simulink model "GridFormingConverter"  (R2024b)
settings: Solver=ode1be  StartTime=0.0  StopTime=simulationTime  FixedStep=gridInverter.vsm.samplingTime  MaxStep=gridInverter.vsm.samplingTime  RelTol=1e-3  AbsTol=1e-3
PreLoadFcn:
  | % Parameterize the model
  | GridFormingConverterInputParameters;
  | GFLParameters;
PostLoadFcn:
  | GridFormingConverterTestCondition;
  | GFLParameters;
undefined symbols (not defined in the file or in its folder): base, ConvCtrl, ConvPlt, DiscIntNeverNeededParam, Discrete, Fault, gcbh, GFMGFLSelect, grid, gridInverter, HMI, localSolverSampleTime, magnitude, PlantSim, scrFactorRg, scrFactorXg, sps, sps_rtmsupport, spsPLL3phModel, transformer, TransmissionLine, Trf
libraries: powerlib_extras x39, ee_lib x21, eeGeneralControl x19, nesl_utility x16, simulink x13, eeTransforms x10, fl_lib x7, spsSecondOrderFilterLib x4, spsabctodq0Lib x4, spsPower3phInstantaneousLib x3, spsMeanLib x2, eeSinGeneratorThreePhase x1
(part 4 of 6)

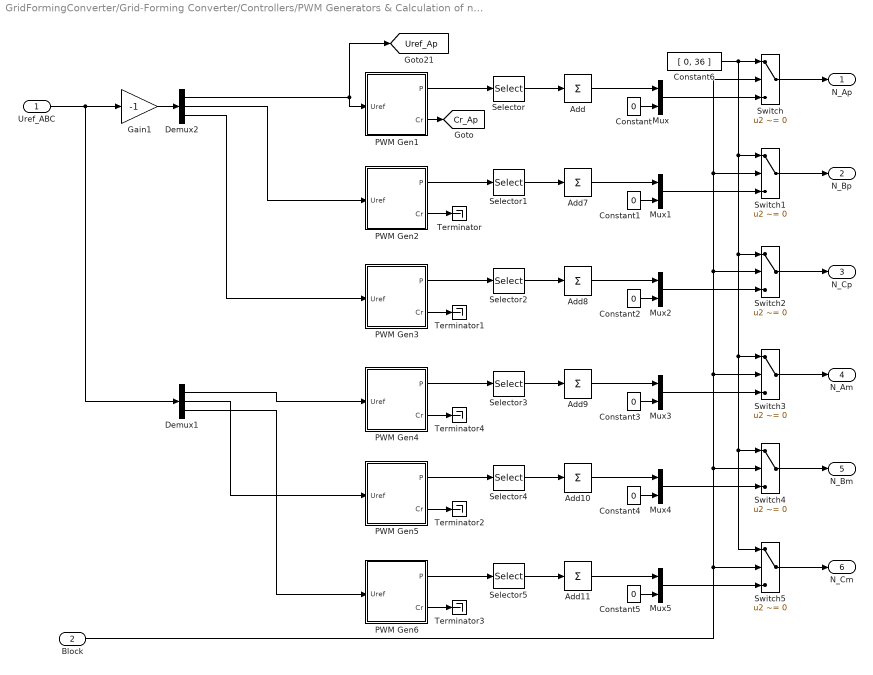
== system GridFormingConverter/Grid-Forming Converter/Controllers/PWM Generators & Calculation of number of inserted modules (Nin) and number of blocked module (Nbl) ==
  Uref_ABC : Inport  PortDimensions=3
  Block : Inport  Port=2
  Add{,7..11} (6 alike) : Sum  Inputs=1
  Constant{,1..5} (6 alike) : Constant  Value=0
  Constant6 : Constant  Value=[ 0, 36 ]
  Demux1 : Demux  Outputs=3
  Demux2 : Demux  Outputs=3
  Gain1 : Gain  Gain=-1
  Mux{,1..5} (6 alike) : Mux  Inputs=2
  PWM Gen1 : Subsystem  mask(PWM generator for half-bridge MMC){n=ConvPlt.Nb_PM, Fc=ConvPlt.Fc, Ts=PlantSim.Ts}
      mask prompts: n "Number of half-bridges"; Fc "Carriers frequency (Hz)"; Ts "Sample time (s)"
      mask init:
      | Tc=1/Fc;
      |         Pc= [ 0:360/n:360-360/n]*pi/180;
      |         Offset=Pc/(2*pi);
      |         Offset_Cr=Pc/(2*pi)*Tc;
      |         p=0;
      |         for m=1:2:2*n
      |             p=p+1;
      |             SelectPulsesPS(m)=p;
      |             SelectPulsesPS(m+1)=p+n;
      |         end
  PWM Gen2 : Subsystem  mask(PWM generator for half-bridge MMC){n=ConvPlt.Nb_PM, Fc=ConvPlt.Fc, Ts=PlantSim.Ts}
      mask prompts: n "Number of half-bridges"; Fc "Carriers frequency (Hz)"; Ts "Sample time (s)"
      mask init: same as GridFormingConverter/Grid-Forming Converter/Controllers/PWM Generators & Calculation of number of inserted modules (Nin) and number of blocked module (Nbl)/PWM Gen1
  PWM Gen3 : Subsystem  mask(PWM generator for half-bridge MMC){n=ConvPlt.Nb_PM, Fc=ConvPlt.Fc, Ts=PlantSim.Ts}
      mask prompts: n "Number of half-bridges"; Fc "Carriers frequency (Hz)"; Ts "Sample time (s)"
      mask init: same as GridFormingConverter/Grid-Forming Converter/Controllers/PWM Generators & Calculation of number of inserted modules (Nin) and number of blocked module (Nbl)/PWM Gen1
  PWM Gen4 : Subsystem  mask(PWM generator for half-bridge MMC){n=ConvPlt.Nb_PM, Fc=ConvPlt.Fc, Ts=PlantSim.Ts}
      mask prompts: n "Number of half-bridges"; Fc "Carriers frequency (Hz)"; Ts "Sample time (s)"
      mask init: same as GridFormingConverter/Grid-Forming Converter/Controllers/PWM Generators & Calculation of number of inserted modules (Nin) and number of blocked module (Nbl)/PWM Gen1
  PWM Gen5 : Subsystem  mask(PWM generator for half-bridge MMC){n=ConvPlt.Nb_PM, Fc=ConvPlt.Fc, Ts=PlantSim.Ts}
      mask prompts: n "Number of half-bridges"; Fc "Carriers frequency (Hz)"; Ts "Sample time (s)"
      mask init: same as GridFormingConverter/Grid-Forming Converter/Controllers/PWM Generators & Calculation of number of inserted modules (Nin) and number of blocked module (Nbl)/PWM Gen1
  PWM Gen6 : Subsystem  mask(PWM generator for half-bridge MMC){n=ConvPlt.Nb_PM, Fc=ConvPlt.Fc, Ts=PlantSim.Ts}
      mask prompts: n "Number of half-bridges"; Fc "Carriers frequency (Hz)"; Ts "Sample time (s)"
      mask init: same as GridFormingConverter/Grid-Forming Converter/Controllers/PWM Generators & Calculation of number of inserted modules (Nin) and number of blocked module (Nbl)/PWM Gen1
  Selector{,1..5} (6 alike) : Selector  InputPortWidth=72  IndexOptions=Index vector (dialog)  Indices=[1:2:71]  OutputSizes=1
  Switch{,1..5} (6 alike) : Switch  Criteria=u2 ~= 0  SaturateOnIntegerOverflow=off  InputSameDT=off
  Terminator{,1..4} (5 alike) : Terminator
  N_Ap : Outport
  N_Bp : Outport  Port=2
  N_Cp : Outport  Port=3
  N_Am : Outport  Port=4
  N_Bm : Outport  Port=5
  N_Cm : Outport  Port=6
  tag scope: Cr_Ap=global, Uref_Ap=global
  wires:
  Demux1/2 -> PWM Gen5/1(Uref)
  Demux1/3 -> PWM Gen6/1(Uref)
  Demux1/1 -> PWM Gen4/1(Uref)
  Demux2/3 -> PWM Gen3/1(Uref)
  PWM Gen1/1(P) -> Selector/1
  PWM Gen2/1(P) -> Selector1/1
  PWM Gen3/1(P) -> Selector2/1
  PWM Gen4/1(P) -> Selector3/1
  PWM Gen5/1(P) -> Selector4/1
  PWM Gen6/1(P) -> Selector5/1
  Mux2/1 -> Switch2/3
  Mux5/1 -> Switch5/3
  Mux4/1 -> Switch4/3
  Mux3/1 -> Switch3/3
  Block/1 -> Switch5/2, Switch4/2, Switch3/2, Switch2/2, Switch1/2, Switch/2
  Add11/1 -> Mux5/1
  Add10/1 -> Mux4/1
  Constant3/1 -> Mux3/2
  Switch5/1 -> N_Cm/1
  Add/1 -> Mux/1
  Switch4/1 -> N_Bm/1
  Switch2/1 -> N_Cp/1
  Constant4/1 -> Mux4/2
  Switch1/1 -> N_Bp/1
  Mux/1 -> Switch/3
  Add8/1 -> Mux2/1
  Add9/1 -> Mux3/1
  Constant2/1 -> Mux2/2
  Constant6/1 -> Switch1/1, Switch2/1, Switch3/1, Switch4/1, Switch5/1, Switch/1
  Mux1/1 -> Switch1/3
  Switch3/1 -> N_Am/1
  Switch/1 -> N_Ap/1
  Constant5/1 -> Mux5/2
  Constant1/1 -> Mux1/2
  Add7/1 -> Mux1/1
  Constant/1 -> Mux/2
  Selector5/1 -> Add11/1
  Selector4/1 -> Add10/1
  Selector3/1 -> Add9/1
  Selector2/1 -> Add8/1
  Selector1/1 -> Add7/1
  Selector/1 -> Add/1
  PWM Gen3/2(Cr) -> Terminator1/1
  PWM Gen1/2(Cr) -> [Cr_Ap]
  Gain1/1 -> Demux2/1
  Demux2/1 -> [Uref_Ap], PWM Gen1/1(Uref)
  Demux2/2 -> PWM Gen2/1(Uref)
  PWM Gen2/2(Cr) -> Terminator/1
  PWM Gen6/2(Cr) -> Terminator3/1
  Uref_ABC/1 -> Demux1/1, Gain1/1
  PWM Gen5/2(Cr) -> Terminator2/1
  PWM Gen4/2(Cr) -> Terminator4/1

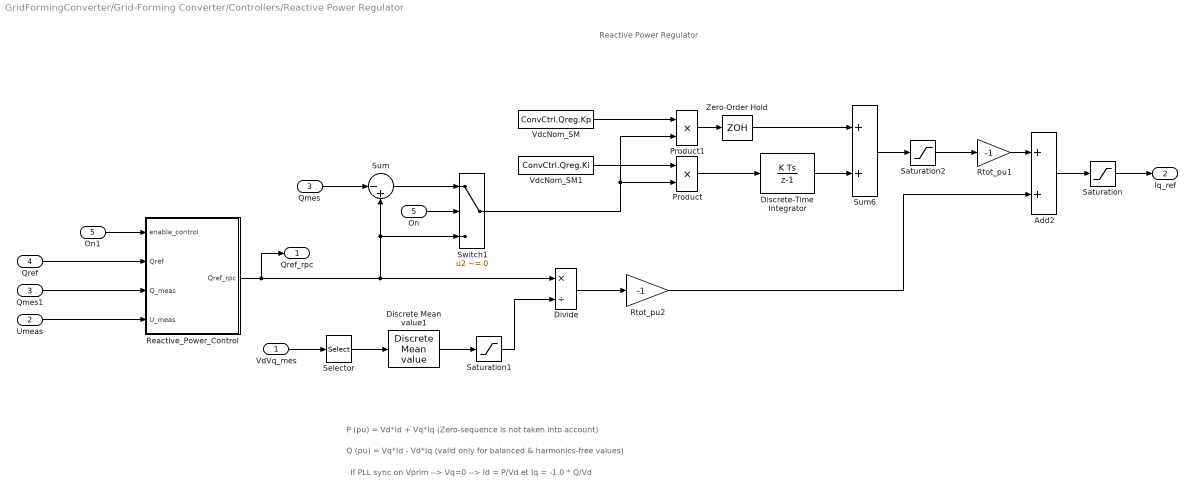
== system GridFormingConverter/Grid-Forming Converter/Controllers/Reactive Power Regulator ==
  note: P (pu) = Vd*Id + Vq*Iq (Zero-sequence is not taken into account)
  note: Q (pu) = Vq*Id - Vd*Iq (valid only for balanced & harmonics-free values)
  note: If PLL sync on Vprim --> Vq=0 --> Id = P/Vd et Iq = -1.0 * Q/Vd
  note: Reactive Power Regulator
  VdVq_mes : Inport  PortDimensions=2
  Umeas : Inport  Port=2  PortDimensions=1
  Qmes : Inport  Port=3  PortDimensions=1
  Qref : Inport  Port=4  PortDimensions=1
  On : Inport  Port=5  PortDimensions=1
  Add2 : Sum
  Discrete Mean value1 : powerlib_extras/Discrete Measurements/Discrete  Mean value  Freq=ConvCtrl.Freq  Vinit=0  Ts=ConvCtrl.Ts
  Discrete-Time Integrator : DiscreteIntegrator  SampleTime=ConvCtrl.Ts  LimitOutput=on  UpperSaturationLimit=ConvCtrl.Qreg.Limits(1)  LowerSaturationLimit=ConvCtrl.Qreg.Limits(2)  ICPrevOutput=DiscIntNeverNeededParam  ICPrevScaledInput=DiscIntNeverNeededParam
  Divide : Product  Inputs=*/
  On1 : InportShadow  Port=5  PortDimensions=1
  Product : Product  RndMeth=Zero
  Product1 : Product  RndMeth=Zero
  Qmes1 : InportShadow  Port=3  PortDimensions=1
  Reactive_Power_Control : Subsystem
  Rtot_pu1 : Gain  Gain=-1  SaturateOnIntegerOverflow=on  OutDataTypeStr=Inherit: Same as input  ParamDataTypeStr=Inherit: Same as input
  Rtot_pu2 : Gain  Gain=-1  SaturateOnIntegerOverflow=on  OutDataTypeStr=Inherit: Same as input  ParamDataTypeStr=Inherit: Same as input
  Saturation : Saturate  UpperLimit=ConvCtrl.Qreg.Limits(1)  LowerLimit=ConvCtrl.Qreg.Limits(2)
  Saturation1 : Saturate  UpperLimit=2  LowerLimit=1e-6
  Saturation2 : Saturate  UpperLimit=ConvCtrl.Qreg.Limits(1)  LowerLimit=ConvCtrl.Qreg.Limits(2)
  Selector : Selector  InputPortWidth=2  IndexOptions=Index vector (dialog)  Indices=[1]  OutputSizes=1
  Sum : Sum  Inputs=|-+
  Sum6 : Sum  InputSameDT=on  SaturateOnIntegerOverflow=on  SampleTime=ConvCtrl.Ts  OutDataTypeStr=Inherit: Same as first input
  Switch1 : Switch  Criteria=u2 ~= 0  Threshold=0.5  OutDataTypeStr=double  SaturateOnIntegerOverflow=off  InputSameDT=off
  VdcNom_SM : Constant  Value=ConvCtrl.Qreg.Kp
  VdcNom_SM1 : Constant  Value=ConvCtrl.Qreg.Ki
  Zero-Order Hold : ZeroOrderHold  SampleTime=ConvCtrl.Ts
  Qref_rpc : Outport
  Iq_ref : Outport  Port=2
  wires:
  Qref/1 -> Reactive_Power_Control/2(Qref)
  Umeas/1 -> Reactive_Power_Control/4(U_meas)
  Qmes1/1 -> Reactive_Power_Control/3(Q_meas)
  On1/1 -> Reactive_Power_Control/1(enable_control)
  Reactive_Power_Control/1(Qref_rpc) -> Sum/2, Switch1/3, Divide/1, Qref_rpc/1
  Qmes/1 -> Sum/1
  VdVq_mes/1 -> Selector/1
  Selector/1 -> Discrete Mean value1/1
  Divide/1 -> Rtot_pu2/1
  Saturation1/1 -> Divide/2
  Discrete Mean value1/1 -> Saturation1/1
  Zero-Order Hold/1 -> Sum6/1
  Discrete-Time Integrator/1 -> Sum6/2
  VdcNom_SM1/1 -> Product/1
  VdcNom_SM/1 -> Product1/1
  Product1/1 -> Zero-Order Hold/1
  Product/1 -> Discrete-Time Integrator/1
  Add2/1 -> Saturation/1
  On/1 -> Switch1/2
  Sum/1 -> Switch1/1
  Switch1/1 -> Product/2, Product1/2
  Sum6/1 -> Saturation2/1
  Rtot_pu1/1 -> Add2/1
  Rtot_pu2/1 -> Add2/2
  Saturation/1 -> Iq_ref/1
  Saturation2/1 -> Rtot_pu1/1

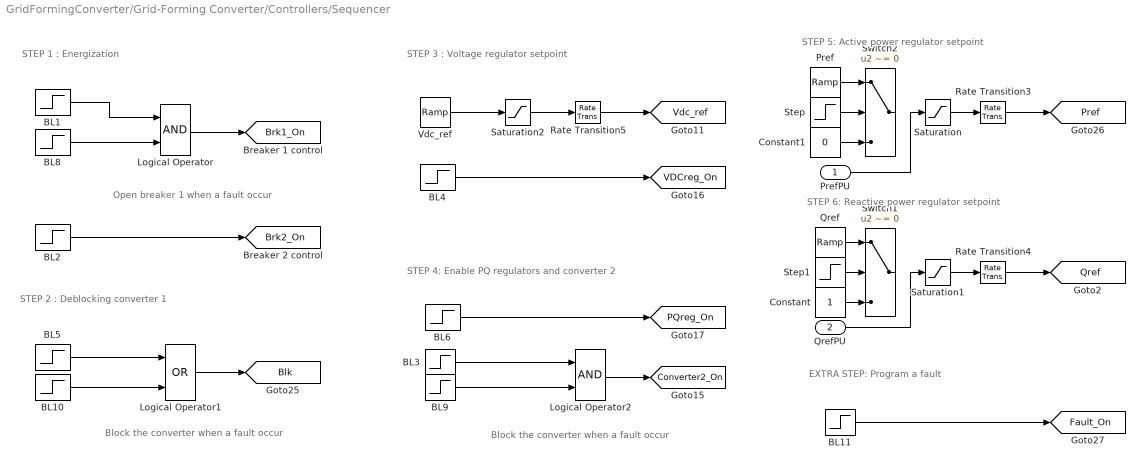
== system GridFormingConverter/Grid-Forming Converter/Controllers/Sequencer ==
  note: EXTRA STEP: Program a fault
  note: STEP 1 : Energization
  note: STEP 2 : Deblocking converter 1
  note: STEP 3 : Voltage regulator setpoint
  note: STEP 5: Active power regulator setpoint
  note: STEP 4: Enable PQ regulators and converter 2
  note: STEP 6: Reactive power regulator setpoint
  note: Block the converter when a fault occur
  note: Block the converter when a fault occur
  note: Open breaker 1 when a fault occur
  PrefPU : Inport
  QrefPU : Inport  Port=2
  BL1 : Step  Time=HMI.Tbrk1_On  SampleTime=PlantSim.Ts
  BL10 : Step  Time=9999  SampleTime=PlantSim.Ts
  BL11 : Step  Time=9999  SampleTime=PlantSim.Ts
  BL2 : Step  Time=HMI.Tbrk2_On  SampleTime=PlantSim.Ts
  BL3 : Step  Time=HMI.Ton_Converter2  SampleTime=PlantSim.Ts
  BL4 : Step  Time=HMI.Ton_VDCreg  SampleTime=ConvCtrl.Ts
  BL5 : Step  Time=HMI.Tdeblock  Before=1  After=0  SampleTime=PlantSim.Ts
  BL6 : Step  Time=HMI.Ton_PQreg  SampleTime=ConvCtrl.Ts
  BL8 : Step  Time=9999  Before=1  After=0  SampleTime=PlantSim.Ts
  BL9 : Step  Time=9999  Before=1  After=0  SampleTime=PlantSim.Ts
  Constant : Constant
  Constant1 : Constant  Value=0
  Logical Operator : Logic  AllPortsSameDT=off  OutDataTypeStr=boolean
  Logical Operator1 : Logic  Operator=OR  AllPortsSameDT=off  OutDataTypeStr=float('double')
  Logical Operator2 : Logic  AllPortsSameDT=off  OutDataTypeStr=boolean
  Pref : simulink/Sources/Ramp  slope=HMI.Slope_Pref  start=HMI.Tramping_Pref  InitialOutput=0
  Qref : simulink/Sources/Ramp  slope=-HMI.Slope_Qref  start=HMI.Tramping_Qref  InitialOutput=0
  Rate Transition3 : RateTransition  OutPortSampleTime=ConvCtrl.Ts
  Rate Transition4 : RateTransition  OutPortSampleTime=ConvCtrl.Ts
  Rate Transition5 : RateTransition  OutPortSampleTime=ConvCtrl.Ts
  Saturation : Saturate  UpperLimit=1*1+0.832*0  LowerLimit=-1
  Saturation1 : Saturate  UpperLimit=ConvCtrl.Qreg.Limits(1)  LowerLimit=ConvCtrl.Qreg.Limits(2)
  Saturation2 : Saturate  UpperLimit=ConvPlt.Vnom_dc  LowerLimit=eps
  Step : Step  Time=Fault.StartTime  Before=1  After=0
  Step1 : Step  Time=Fault.StartTime  Before=1  After=0
  Switch1 : Switch  Criteria=u2 ~= 0  SaturateOnIntegerOverflow=off  InputSameDT=off
  Switch2 : Switch  Criteria=u2 ~= 0  SaturateOnIntegerOverflow=off  InputSameDT=off
  "Vdc_ref " : simulink/Sources/Ramp  slope=HMI.Slope_Vdc_ref  start=HMI.Tramping_Vdc_ref  InitialOutput=Trf.Vsecondary *1.37*ConvPlt.Vnom_dc
  tag scope: Blk=global, Brk1_On=global, Brk2_On=global, Converter2_On=global, Fault_On=global, PQreg_On=global, Pref=global, Qref=global, VDCreg_On=global, Vdc_ref=global
  wires:
  Constant1/1 -> Switch2/3
  Constant/1 -> Switch1/3
  Pref/1 -> Switch2/1
  Qref/1 -> Switch1/1
  Step1/1 -> Switch1/2
  Step/1 -> Switch2/2
  BL11/1 -> [Fault_On]
  BL10/1 -> Logical Operator1/2
  BL5/1 -> Logical Operator1/1
  Logical Operator1/1 -> [Blk]
  Logical Operator2/1 -> [Converter2_On]
  BL3/1 -> Logical Operator2/1
  BL9/1 -> Logical Operator2/2
  BL1/1 -> Logical Operator/1
  Logical Operator/1 -> [Brk1_On]
  BL8/1 -> Logical Operator/2
  BL2/1 -> [Brk2_On]
  "Vdc_ref "/1 -> Saturation2/1
  BL6/1 -> [PQreg_On]
  BL4/1 -> [VDCreg_On]
  Rate Transition5/1 -> [Vdc_ref]
  Rate Transition4/1 -> [Qref]
  Rate Transition3/1 -> [Pref]
  Saturation/1 -> Rate Transition3/1
  QrefPU/1 -> Saturation1/1
  PrefPU/1 -> Saturation/1
  Saturation1/1 -> Rate Transition4/1
  Saturation2/1 -> Rate Transition5/1

== system GridFormingConverter/Grid-Forming Converter/Grid-Forming Converter Control/Current Limiting ==
  In Bus Element : Inport  PortName=measure  Element=Igd
  In Bus Element1 : Inport  PortName=measure  Element=Igq
  In Bus Element2 : Inport  Port=2  PortName=reactiveControl  Element=Vmd
  In Bus Element4 : Inport  Port=2  PortName=reactiveControl  Element=Vmq
  CurrentLimitingMethod : Subsystem  Variant=on  VariantControlMode=label  VariantControl=Choice  LabelModeActiveChoice=virimp
  Subtract : Sum  Inputs=+-
  Subtract1 : Sum  Inputs=-+
  Out Bus Element : Outport  PortName=currentLimiting  Element=Vmd
  Out Bus Element1 : Outport  PortName=currentLimiting  Element=Vmq
  Out Bus Element2 : Outport  PortName=currentLimiting  Element=Idmax
  Out Bus Element3 : Outport  PortName=currentLimiting  Element=Iqmax
  wires:
  In Bus Element2/1 -> Subtract/1
  In Bus Element1/1 -> CurrentLimitingMethod/2(Igq)
  In Bus Element4/1 -> Subtract1/2
  Subtract/1 -> Out Bus Element/1
  Subtract1/1 -> Out Bus Element1/1
  In Bus Element/1 -> CurrentLimitingMethod/1(Igd)  "Q"
  CurrentLimitingMethod/1(delVd) -> Subtract/2
  CurrentLimitingMethod/2(delVq) -> Subtract1/1
  CurrentLimitingMethod/3(Idmax) -> Out Bus Element2/1
  CurrentLimitingMethod/4(Iqmax) -> Out Bus Element3/1

== system GridFormingConverter/Grid-Forming Converter/Grid-Forming Converter Control/Grid Voltage Reactive Power Support ==
  In Bus Element1 : Inport  PortName=measure  Element=Vgd
  In Bus Element3 : Inport  PortName=measure  Element=Vgq
  In Bus Element2 : Inport  PortName=measure  Element=Igd
  In Bus Element4 : Inport  PortName=measure  Element=Igq
  PrefInput : Inport  Port=2
  QrefInput : Inport  Port=3
  Modifying Active Power Reference : Subsystem
  Modifying Reactive Power Reference : Subsystem
  Rate Transition{,1..5} (6 alike) : RateTransition
  Pref : Outport
  Qref : Outport  Port=2
  wires:
  PrefInput/1 -> Modifying Active Power Reference/1(PrefInput)
  In Bus Element2/1 -> Modifying Active Power Reference/3(Igd)
  In Bus Element4/1 -> Modifying Active Power Reference/4(Igq)
  In Bus Element3/1 -> Rate Transition2/1
  QrefInput/1 -> Rate Transition3/1
  Modifying Reactive Power Reference/1(PrefNew) -> Rate Transition4/1
  Modifying Reactive Power Reference/2(QrefNew) -> Rate Transition5/1
  In Bus Element1/1 -> Rate Transition/1
  Modifying Active Power Reference/1(Pref) -> Rate Transition1/1
  Rate Transition2/1 -> Modifying Reactive Power Reference/2(Vgq)
  Rate Transition3/1 -> Modifying Reactive Power Reference/3(Qref)
  Rate Transition1/1 -> Modifying Reactive Power Reference/4(Pref)
  Rate Transition4/1 -> Pref/1
  Rate Transition5/1 -> Qref/1
  Rate Transition/1 -> Modifying Reactive Power Reference/1(Vgd), Modifying Active Power Reference/2(Vd)

== system GridFormingConverter/Grid-Forming Converter/Grid-Forming Converter Control/Measurement ==
  Vgabcc : Inport
  Igabc : Inport  Port=2
  Angle : Inport  Port=3
  Frequency Measurement : Subsystem
  Gain1 : Gain  Gain=1/power
  Gain2 : Gain  Gain=1/power
  Gain3 : Gain  Gain=1/(gridLineVoltage*sqrt(2/3))
  Gain4 : Gain  Gain=1/(gridLineVoltage*sqrt(2/3))
  Gain5 : Gain  Gain=1/(power/(sqrt(3)*gridLineVoltage)*sqrt(2))
  Gain6 : Gain  Gain=1/(power/(sqrt(3)*gridLineVoltage)*sqrt(2))
  Power Measurement (Three-Phase) : eePowerMeasurement/Power Measurement (Three-Phase)  LabelModeActiveChoice=Discrete  F=powerFreq  K=[1]  Seq=Positive  Ts=measSampleTime
  abc2dq : Subsystem
  Out Bus Element : Outport  PortName=measure  Element=P
  Out Bus Element1 : Outport  PortName=measure  Element=Q
  Out Bus Element2 : Outport  PortName=measure  Element=Vgd
  Out Bus Element3 : Outport  PortName=measure  Element=Vgq
  Out Bus Element4 : Outport  PortName=measure  Element=Igd
  Out Bus Element5 : Outport  PortName=measure  Element=Igq
  Out Bus Element6 : Outport  PortName=measure  Element=fgrid
  Pmeas : Outport  Port=2
  Qmeas : Outport  Port=3
  fmeas : Outport  Port=4
  wires:
  Vgabcc/1 -> abc2dq/3(Vgabc), Frequency Measurement/1(Vabc), Power Measurement (Three-Phase)/1  "Vabc"
  Angle/1 -> abc2dq/2(Angle)
  Power Measurement (Three-Phase)/1 -> Gain2/1
  Igabc/1 -> abc2dq/1(Igabc), Power Measurement (Three-Phase)/2  "Iabc"
  Power Measurement (Three-Phase)/2 -> Gain1/1
  Gain2/1 -> Pmeas/1, Out Bus Element/1  "Pmeas"
  Gain1/1 -> Qmeas/1, Out Bus Element1/1  "Qmeas"
  abc2dq/1(Vgd) -> Gain4/1
  abc2dq/2(Vgq) -> Gain3/1
  abc2dq/3(Igd) -> Gain5/1
  abc2dq/4(Igq) -> Gain6/1
  Gain3/1 -> Out Bus Element3/1  "Vgq"
  Gain4/1 -> Out Bus Element2/1  "Vgd"
  Gain5/1 -> Out Bus Element4/1  "Igd"
  Gain6/1 -> Out Bus Element5/1  "Igq"
  Frequency Measurement/1(freq) -> Out Bus Element6/1, fmeas/1

== system GridFormingConverter/Grid-Forming Converter/Grid-Forming Converter Control/Power Control ==
  note: Reactive Power Control
  note: Active Power Control
  In Bus Element2 : Inport  PortName=measure  Element=P
  In Bus Element3 : Inport  PortName=measure  Element=Q
  In Bus Element1 : Inport  PortName=measure  Element=fgrid
  Pref : Inport  Port=2
  Qref : Inport  Port=3
  ActivePowerControl : Subsystem  Variant=on  VariantControlMode=label  VariantControl=Choice  LabelModeActiveChoice=vsm
  ReactiveControl : Subsystem
  Out Bus Element : Outport  PortName=reactiveControl  Element=Vmd
  Out Bus Element1 : Outport  PortName=reactiveControl  Element=Vmq
  Out Bus Element6 : Outport  Port=2  PortName=activeControl  Element=angle
  Out Bus Element4 : Outport  Port=2  PortName=activeControl  Element=w
  angle : Outport  Port=3
  wires:
  ActivePowerControl/2(w) -> Out Bus Element4/1
  In Bus Element3/1 -> ReactiveControl/2(Qmeas)
  ActivePowerControl/1(Theta) -> angle/1, Out Bus Element6/1
  ReactiveControl/1(Vmd) -> Out Bus Element/1
  ReactiveControl/2(Vmq) -> Out Bus Element1/1
  Pref/1 -> ActivePowerControl/1(Pref)  "Q"
  Qref/1 -> ReactiveControl/1(Qref)  "Q"
  In Bus Element2/1 -> ActivePowerControl/2(Pmeas)
  In Bus Element1/1 -> ActivePowerControl/3(fgrid)

== system GridFormingConverter/Grid-Forming Converter/Grid-Forming Converter Control/VoltageCurrentControl ==
  In Bus Element : Inport  PortName=currentLimiting  Element=Vmd
  In Bus Element1 : Inport  PortName=currentLimiting  Element=Vmq
  In Bus Element6 : Inport  PortName=currentLimiting  Element=Idmax
  In Bus Element7 : Inport  PortName=currentLimiting  Element=Iqmax
  Bus Element In6 : Inport  Port=2  PortName=activeControl  Element=w
  Bus Element In1 : Inport  Port=2  PortName=activeControl  Element=angle
  In Bus Element2 : Inport  Port=3  PortName=measure  Element=Vgd
  In Bus Element3 : Inport  Port=3  PortName=measure  Element=Vgq
  In Bus Element4 : Inport  Port=3  PortName=measure  Element=Igd
  In Bus Element5 : Inport  Port=3  PortName=measure  Element=Igq
  Controller : Subsystem
  Modulation Signal : Subsystem
  mabc : Outport
  wires:
  Controller/2(Vq) -> Modulation Signal/2(Vq)
  Modulation Signal/1(mabc) -> mabc/1
  Controller/1(Vd) -> Modulation Signal/1(Vd)
  In Bus Element4/1 -> Controller/6(Id)
  In Bus Element5/1 -> Controller/7(Iq)
  In Bus Element6/1 -> Controller/8(Idmax)
  In Bus Element7/1 -> Controller/9(Iqmax)
  In Bus Element2/1 -> Controller/4(Vsd)
  In Bus Element3/1 -> Controller/5(Vsq)
  Bus Element In6/1 -> Controller/1(Angfreq)
  In Bus Element/1 -> Controller/2(Vgdref)
  In Bus Element1/1 -> Controller/3(Vgqref)
  Bus Element In1/1 -> Modulation Signal/3(Angle)

== system GridFormingConverter/Grid-Forming Converter/Grid-Forming Converter Power Circuit/Filter & Sensor ==
  Current Sensor (Three-Phase) : ee_lib/Sensors & Transducers/Current Sensor (Three-Phase)
  Electrical Reference1 : fl_lib/Electrical/Electrical Elements/Electrical Reference
  Low-Pass Filter (Discrete or Continuous)1 : eeGeneralControl/Low-Pass Filter (Discrete or Continuous)  K=1  T=1/(200*gridInverter.frequency)  B=inf  A=-inf  init_option=Specify as parameter  x0=0  Ts=gridInverter.controller.VoltageControlSampleTime
  Low-Pass Filter (Discrete or Continuous)2 : eeGeneralControl/Low-Pass Filter (Discrete or Continuous)  K=1  T=1/(200*gridInverter.frequency)  B=inf  A=-inf  init_option=Specify as parameter  x0=0  Ts=gridInverter.controller.VoltageControlSampleTime
  Neutral Port (Three-Phase) : ee_lib/Connectors & References/Neutral Port (Three-Phase)  G_parasitic=1e-12 1/Ohm
      settings: InternalSimscapePortConfiguration="{\"Bottom\":[],\"Left\":[{\"id\":\"N\",\"label\":\"~\",\"type\":\"foundation.electrical.three_phase\"}],\"Right\":[{\"id\":\"n\",\"label\":\"n\",\"type\":\"foundation.electrical.electrical\"}],\"Top\":[]}"
  PS-Simulink Converter : nesl_utility/PS-Simulink Converter  PhysicalDomain=network_engine_domain  SubClassName=ps_output  LeftPortType=input  RightPortType=output  PseudoPeriodic=off  Frequencies=[]  VectorFormat=inherit  Unit=inherit  AffineConversion=off
  PS-Simulink Converter1 : nesl_utility/PS-Simulink Converter  PhysicalDomain=network_engine_domain  SubClassName=ps_output  LeftPortType=input  RightPortType=output  PseudoPeriodic=off  Frequencies=[]  VectorFormat=inherit  Unit=inherit  AffineConversion=off
  Phase Voltage Sensor (Three-Phase) : ee_lib/Sensors & Transducers/Phase Voltage Sensor (Three-Phase)
  RLC (Three-Phase) : ee_lib/Passive/RLC Assemblies/RLC (Three-Phase)  port_option=ee.enum.threePhasePort.composite  component_structure=ee.enum.rlc.structure.SeriesRL  R=gridInverter.lineResistance Ohm  L=gridInverter.L H  C=1e-6 F  R_parasitic=0 Ohm  G_parasitic=0 1/Ohm  IL_specify=off  IL_priority=High  IL=[0, 0, 0] A  IL_nominal_specify=off  IL_nominal_value=1  IL_nominal_unit=A  VC_specify=off  VC_priority=High  VC=[0, 0, 0] V  VC_nominal_specify=off  VC_nominal_value=1  VC_nominal_unit=V
      settings: InternalSimscapePortConfiguration="{\"Bottom\":[],\"Left\":[{\"id\":\"N1\",\"label\":\"~1\",\"type\":\"foundation.electrical.three_phase\"}],\"Right\":[{\"id\":\"N2\",\"label\":\"~2\",\"type\":\"foundation.electrical.three_phase\"}],\"Top\":[]}"
  Inabc : PMIOPort  Side=Left
  Opabc : PMIOPort  Port=2  Side=Right
  Iabc : Outport
  Vabc : Outport  Port=2
  wires:
  PS-Simulink Converter1/1 -> Low-Pass Filter (Discrete or Continuous)1/1
  Low-Pass Filter (Discrete or Continuous)2/1 -> Iabc/1
  PS-Simulink Converter/1 -> Low-Pass Filter (Discrete or Continuous)2/1
  Low-Pass Filter (Discrete or Continuous)1/1 -> Vabc/1
  connections:
  PS-Simulink Converter1/LConn1 -- Phase Voltage Sensor (Three-Phase)/RConn1
  Current Sensor (Three-Phase)/RConn2 -- RLC (Three-Phase)/LConn1
  Current Sensor (Three-Phase)/LConn1 -- Inabc/RConn1
  PS-Simulink Converter/LConn1 -- Current Sensor (Three-Phase)/RConn1
  Phase Voltage Sensor (Three-Phase)/LConn1 -- Opabc/RConn1 -- RLC (Three-Phase)/RConn1
  Phase Voltage Sensor (Three-Phase)/RConn2 -- Neutral Port (Three-Phase)/LConn1
  Electrical Reference1/LConn1 -- Neutral Port (Three-Phase)/RConn1

== system GridFormingConverter/Grid-Forming Converter/BusCalculations/Measurement Unit (Phasor Computation)/Discrete Fourier(A) ==
  note: Discrete Fourier
  note: Pierre Giroux, Gilbert Sybille
      | Power System Simulation Laboratory
      | IREQ, Hydro-Quebc
  In : Inport
  Demux : Demux  Outputs=2
      settings: DisplayOption=none
  Discrete Mean value1 : powerlib_extras/Discrete Measurements/Discrete  Mean value  Freq=Freq  Vinit=Real_Init  Ts=Ts
  Discrete Mean value2 : powerlib_extras/Discrete Measurements/Discrete  Mean value  Freq=Freq  Vinit=Imag_Init  Ts=Ts
  Gain : Gain  Gain=2*pi*n*Freq  SaturateOnIntegerOverflow=on  OutDataTypeStr=Inherit: Same as input  ParamDataTypeStr=Inherit: Same as input
  Gain1 : Gain  Gain=k  SaturateOnIntegerOverflow=on  OutDataTypeStr=Inherit: Same as input  ParamDataTypeStr=Inherit: Same as input
  Mux : Mux  Inputs=2
  Product : Product  InputSameDT=on  SaturateOnIntegerOverflow=on  OutDataTypeStr=Inherit: Same as first input
  Real-Imag to Complex : RealImagToComplex
  Trigonometric Function : Trigonometry
  Trigonometric Function1 : Trigonometry  Operator=cos
  t : DigitalClock  SampleTime=Ts
  Fund : Outport
  wires:
  Real-Imag to Complex/1 -> Fund/1
  Discrete Mean value2/1 -> Real-Imag to Complex/2  "Imag"
  Discrete Mean value1/1 -> Real-Imag to Complex/1  "Real"
  t/1 -> Gain/1
  Gain/1 -> Trigonometric Function/1, Trigonometric Function1/1
  Trigonometric Function/1 -> Mux/1
  Trigonometric Function1/1 -> Mux/2
  Mux/1 -> Gain1/1
  In/1 -> Product/1
  Gain1/1 -> Product/2
  Product/1 -> Demux/1
  Demux/1 -> Discrete Mean value1/1
  Demux/2 -> Discrete Mean value2/1

== system GridFormingConverter/Grid-Forming Converter/BusCalculations/Measurement Unit (Phasor Computation)/Discrete Fourier(A)  ==
  note: Pierre Giroux, Gilbert Sybille
      | Power System Simulation Laboratory
      | IREQ, Hydro-Quebc
  note: Discrete Fourier
  In : Inport
  Demux : Demux  Outputs=2
      settings: DisplayOption=none
  Discrete Mean value1 : powerlib_extras/Discrete Measurements/Discrete  Mean value  Freq=Freq  Vinit=Real_Init  Ts=Ts
  Discrete Mean value2 : powerlib_extras/Discrete Measurements/Discrete  Mean value  Freq=Freq  Vinit=Imag_Init  Ts=Ts
  Gain : Gain  Gain=2*pi*n*Freq  SaturateOnIntegerOverflow=on  OutDataTypeStr=Inherit: Same as input  ParamDataTypeStr=Inherit: Same as input
  Gain1 : Gain  Gain=k  SaturateOnIntegerOverflow=on  OutDataTypeStr=Inherit: Same as input  ParamDataTypeStr=Inherit: Same as input
  Mux : Mux  Inputs=2
  Product : Product  InputSameDT=on  SaturateOnIntegerOverflow=on  OutDataTypeStr=Inherit: Same as first input
  Real-Imag to Complex : RealImagToComplex
  Trigonometric Function : Trigonometry
  Trigonometric Function1 : Trigonometry  Operator=cos
  t : DigitalClock  SampleTime=Ts
  Fund : Outport
  wires:
  Demux/2 -> Discrete Mean value2/1
  Demux/1 -> Discrete Mean value1/1
  Product/1 -> Demux/1
  Gain1/1 -> Product/2
  In/1 -> Product/1
  Mux/1 -> Gain1/1
  Trigonometric Function1/1 -> Mux/2
  Trigonometric Function/1 -> Mux/1
  Gain/1 -> Trigonometric Function1/1, Trigonometric Function/1
  t/1 -> Gain/1
  Discrete Mean value1/1 -> Real-Imag to Complex/1  "Real"
  Discrete Mean value2/1 -> Real-Imag to Complex/2  "Imag"
  Real-Imag to Complex/1 -> Fund/1

== system GridFormingConverter/Grid-Forming Converter/BusCalculations/Measurement Unit (Phasor Computation)/Discrete Fourier(B) ==
  note: Pierre Giroux, Gilbert Sybille
      | Power System Simulation Laboratory
      | IREQ, Hydro-Quebc
  note: Discrete Fourier
  In : Inport
  Demux : Demux  Outputs=2
      settings: DisplayOption=none
  Discrete Mean value1 : powerlib_extras/Discrete Measurements/Discrete  Mean value  Freq=Freq  Vinit=Real_Init  Ts=Ts
  Discrete Mean value2 : powerlib_extras/Discrete Measurements/Discrete  Mean value  Freq=Freq  Vinit=Imag_Init  Ts=Ts
  Gain : Gain  Gain=2*pi*n*Freq  SaturateOnIntegerOverflow=on  OutDataTypeStr=Inherit: Same as input  ParamDataTypeStr=Inherit: Same as input
  Gain1 : Gain  Gain=k  SaturateOnIntegerOverflow=on  OutDataTypeStr=Inherit: Same as input  ParamDataTypeStr=Inherit: Same as input
  Mux : Mux  Inputs=2
  Product : Product  InputSameDT=on  SaturateOnIntegerOverflow=on  OutDataTypeStr=Inherit: Same as first input
  Real-Imag to Complex : RealImagToComplex
  Trigonometric Function : Trigonometry
  Trigonometric Function1 : Trigonometry  Operator=cos
  t : DigitalClock  SampleTime=Ts
  Fund : Outport
  wires:
  Demux/2 -> Discrete Mean value2/1
  Demux/1 -> Discrete Mean value1/1
  Product/1 -> Demux/1
  Gain1/1 -> Product/2
  In/1 -> Product/1
  Mux/1 -> Gain1/1
  Trigonometric Function1/1 -> Mux/2
  Trigonometric Function/1 -> Mux/1
  Gain/1 -> Trigonometric Function1/1, Trigonometric Function/1
  t/1 -> Gain/1
  Discrete Mean value1/1 -> Real-Imag to Complex/1  "Real"
  Discrete Mean value2/1 -> Real-Imag to Complex/2  "Imag"
  Real-Imag to Complex/1 -> Fund/1

== system GridFormingConverter/Grid-Forming Converter/BusCalculations/Measurement Unit (Phasor Computation)/Discrete Fourier(B)  ==
  note: Discrete Fourier
  note: Pierre Giroux, Gilbert Sybille
      | Power System Simulation Laboratory
      | IREQ, Hydro-Quebc
  In : Inport
  Demux : Demux  Outputs=2
      settings: DisplayOption=none
  Discrete Mean value1 : powerlib_extras/Discrete Measurements/Discrete  Mean value  Freq=Freq  Vinit=Real_Init  Ts=Ts
  Discrete Mean value2 : powerlib_extras/Discrete Measurements/Discrete  Mean value  Freq=Freq  Vinit=Imag_Init  Ts=Ts
  Gain : Gain  Gain=2*pi*n*Freq  SaturateOnIntegerOverflow=on  OutDataTypeStr=Inherit: Same as input  ParamDataTypeStr=Inherit: Same as input
  Gain1 : Gain  Gain=k  SaturateOnIntegerOverflow=on  OutDataTypeStr=Inherit: Same as input  ParamDataTypeStr=Inherit: Same as input
  Mux : Mux  Inputs=2
  Product : Product  InputSameDT=on  SaturateOnIntegerOverflow=on  OutDataTypeStr=Inherit: Same as first input
  Real-Imag to Complex : RealImagToComplex
  Trigonometric Function : Trigonometry
  Trigonometric Function1 : Trigonometry  Operator=cos
  t : DigitalClock  SampleTime=Ts
  Fund : Outport
  wires:
  Real-Imag to Complex/1 -> Fund/1
  Discrete Mean value2/1 -> Real-Imag to Complex/2  "Imag"
  Discrete Mean value1/1 -> Real-Imag to Complex/1  "Real"
  t/1 -> Gain/1
  Gain/1 -> Trigonometric Function/1, Trigonometric Function1/1
  Trigonometric Function/1 -> Mux/1
  Trigonometric Function1/1 -> Mux/2
  Mux/1 -> Gain1/1
  In/1 -> Product/1
  Gain1/1 -> Product/2
  Product/1 -> Demux/1
  Demux/1 -> Discrete Mean value1/1
  Demux/2 -> Discrete Mean value2/1

== system GridFormingConverter/Grid-Forming Converter/BusCalculations/Measurement Unit (Phasor Computation)/Discrete Fourier(C) ==
  note: Discrete Fourier
  note: Pierre Giroux, Gilbert Sybille
      | Power System Simulation Laboratory
      | IREQ, Hydro-Quebc
  In : Inport
  Demux : Demux  Outputs=2
      settings: DisplayOption=none
  Discrete Mean value1 : powerlib_extras/Discrete Measurements/Discrete  Mean value  Freq=Freq  Vinit=Real_Init  Ts=Ts
  Discrete Mean value2 : powerlib_extras/Discrete Measurements/Discrete  Mean value  Freq=Freq  Vinit=Imag_Init  Ts=Ts
  Gain : Gain  Gain=2*pi*n*Freq  SaturateOnIntegerOverflow=on  OutDataTypeStr=Inherit: Same as input  ParamDataTypeStr=Inherit: Same as input
  Gain1 : Gain  Gain=k  SaturateOnIntegerOverflow=on  OutDataTypeStr=Inherit: Same as input  ParamDataTypeStr=Inherit: Same as input
  Mux : Mux  Inputs=2
  Product : Product  InputSameDT=on  SaturateOnIntegerOverflow=on  OutDataTypeStr=Inherit: Same as first input
  Real-Imag to Complex : RealImagToComplex
  Trigonometric Function : Trigonometry
  Trigonometric Function1 : Trigonometry  Operator=cos
  t : DigitalClock  SampleTime=Ts
  Fund : Outport
  wires:
  Real-Imag to Complex/1 -> Fund/1
  Discrete Mean value2/1 -> Real-Imag to Complex/2  "Imag"
  Discrete Mean value1/1 -> Real-Imag to Complex/1  "Real"
  t/1 -> Gain/1
  Gain/1 -> Trigonometric Function/1, Trigonometric Function1/1
  Trigonometric Function/1 -> Mux/1
  Trigonometric Function1/1 -> Mux/2
  Mux/1 -> Gain1/1
  In/1 -> Product/1
  Gain1/1 -> Product/2
  Product/1 -> Demux/1
  Demux/1 -> Discrete Mean value1/1
  Demux/2 -> Discrete Mean value2/1

== system GridFormingConverter/Grid-Forming Converter/BusCalculations/Measurement Unit (Phasor Computation)/Discrete Fourier(C)  ==
  note: Pierre Giroux, Gilbert Sybille
      | Power System Simulation Laboratory
      | IREQ, Hydro-Quebc
  note: Discrete Fourier
  In : Inport
  Demux : Demux  Outputs=2
      settings: DisplayOption=none
  Discrete Mean value1 : powerlib_extras/Discrete Measurements/Discrete  Mean value  Freq=Freq  Vinit=Real_Init  Ts=Ts
  Discrete Mean value2 : powerlib_extras/Discrete Measurements/Discrete  Mean value  Freq=Freq  Vinit=Imag_Init  Ts=Ts
  Gain : Gain  Gain=2*pi*n*Freq  SaturateOnIntegerOverflow=on  OutDataTypeStr=Inherit: Same as input  ParamDataTypeStr=Inherit: Same as input
  Gain1 : Gain  Gain=k  SaturateOnIntegerOverflow=on  OutDataTypeStr=Inherit: Same as input  ParamDataTypeStr=Inherit: Same as input
  Mux : Mux  Inputs=2
  Product : Product  InputSameDT=on  SaturateOnIntegerOverflow=on  OutDataTypeStr=Inherit: Same as first input
  Real-Imag to Complex : RealImagToComplex
  Trigonometric Function : Trigonometry
  Trigonometric Function1 : Trigonometry  Operator=cos
  t : DigitalClock  SampleTime=Ts
  Fund : Outport
  wires:
  Demux/2 -> Discrete Mean value2/1
  Demux/1 -> Discrete Mean value1/1
  Product/1 -> Demux/1
  Gain1/1 -> Product/2
  In/1 -> Product/1
  Mux/1 -> Gain1/1
  Trigonometric Function1/1 -> Mux/2
  Trigonometric Function/1 -> Mux/1
  Gain/1 -> Trigonometric Function1/1, Trigonometric Function/1
  t/1 -> Gain/1
  Discrete Mean value1/1 -> Real-Imag to Complex/1  "Real"
  Discrete Mean value2/1 -> Real-Imag to Complex/2  "Imag"
  Real-Imag to Complex/1 -> Fund/1

== system GridFormingConverter/Grid-Forming Converter/Controllers/Current Regulator (Ireg)/PI regulator with anti-windup D ==
  note: Anti-windup mechanism: Method of conditionnal integration
      |
      | The integration is suspended if saturation occurs and the
      | control error is of the same sign as the control signal.
      |
      | [1] L.Rundqwist, "Anti-Reset Windup for PID Controllers," Ph.D. Thesis TRFT-1033,
      | Departement of Automatic Control, Lund Institute of Technology, Lund, Sweeden, 1991.
  Error : Inport  SampleTime=Ts
  Compare To Zero : simulink/Logic and Bit Operations/Compare To Zero  relop=>  OutDataTypeStr=uint8  ZeroCross=off
  Compare To Zero1 : simulink/Logic and Bit Operations/Compare To Zero  relop=<  OutDataTypeStr=uint8  ZeroCross=off
  Constant : Constant  Value=0
  Constant1 : Constant  Value=UpperLimit
  Constant3 : Constant  Value=LowerLimit
  Discrete-Time Integrator : DiscreteIntegrator  IntegratorMethod=Integration: Trapezoidal  InitialCondition=Init  SampleTime=Ts  LimitOutput=on  UpperSaturationLimit=UpperLimit  LowerSaturationLimit=LowerLimit  ShowStatePort=on  ICPrevOutput=DiscIntNeverNeededParam  ICPrevScaledInput=DiscIntNeverNeededParam
  Kp4 : Gain  Gain=Kp  SaturateOnIntegerOverflow=on  SampleTime=Ts  OutDataTypeStr=Inherit: Same as input  ParamDataTypeStr=Inherit: Same as input
  Kp5 : Gain  Gain=Ki  SaturateOnIntegerOverflow=on  SampleTime=Ts  OutDataTypeStr=Inherit: Same as input  ParamDataTypeStr=Inherit: Same as input
  Logical Operator : Logic  AllPortsSameDT=off  OutDataTypeStr=boolean
  Logical Operator1 : Logic  AllPortsSameDT=off  OutDataTypeStr=boolean
  Logical Operator2 : Logic  Operator=OR  AllPortsSameDT=off  OutDataTypeStr=boolean
  Relational Operator : RelationalOperator  OutDataTypeStr=boolean  InputSameDT=off
  Relational Operator1 : RelationalOperator  Operator=<=  OutDataTypeStr=boolean  InputSameDT=off
  Saturation2 : Saturate  UpperLimit=UpperLimit  LowerLimit=LowerLimit  SampleTime=Ts
  Sum1 : Sum  InputSameDT=on  SaturateOnIntegerOverflow=on  SampleTime=Ts  OutDataTypeStr=Inherit: Same as first input
  Sum6 : Sum  InputSameDT=on  SaturateOnIntegerOverflow=on  SampleTime=Ts  OutDataTypeStr=Inherit: Same as first input
  Switch : Switch  Criteria=u2 > Threshold  SaturateOnIntegerOverflow=off  InputSameDT=off
  Zero-Order Hold : ZeroOrderHold  SampleTime=Ts
  Out : Outport  SampleTime=Ts  InitialOutput=0
  wires:
  Kp5/1 -> Switch/3
  Switch/1 -> Discrete-Time Integrator/1
  Saturation2/1 -> Out/1
  Discrete-Time Integrator/1 -> Sum6/2
  Kp4/1 -> Zero-Order Hold/1
  Sum6/1 -> Saturation2/1
  Error/1 -> Kp5/1, Kp4/1, Compare To Zero/1, Compare To Zero1/1
  Compare To Zero1/1 -> Logical Operator1/2  "Error_is_negative"
  Logical Operator1/1 -> Logical Operator2/2
  Logical Operator/1 -> Logical Operator2/1
  Compare To Zero/1 -> Logical Operator/2  "Error_is_positive"
  Constant3/1 -> Relational Operator1/2
  Constant1/1 -> Relational Operator/2
  Relational Operator1/1 -> Logical Operator1/1  "LowerLimit_Is_Reached"
  Relational Operator/1 -> Logical Operator/1  "UpperLimit_is_Reached"
  Logical Operator2/1 -> Switch/2
  Sum1/1 -> Relational Operator/1, Relational Operator1/1
  Discrete-Time Integrator/State -> Sum1/1
  Zero-Order Hold/1 -> Sum6/1, Sum1/2
  Constant/1 -> Switch/1

== system GridFormingConverter/Grid-Forming Converter/Controllers/Current Regulator (Ireg)/PI regulator with anti-windup Q ==
  note: Anti-windup mechanism: Method of conditionnal integration
      |
      | The integration is suspended if saturation occurs and the
      | control error is of the same sign as the control signal.
      |
      | [1] L.Rundqwist, "Anti-Reset Windup for PID Controllers," Ph.D. Thesis TRFT-1033,
      | Departement of Automatic Control, Lund Institute of Technology, Lund, Sweeden, 1991.
  Error : Inport  SampleTime=Ts
  Compare To Zero : simulink/Logic and Bit Operations/Compare To Zero  relop=>  OutDataTypeStr=uint8  ZeroCross=off
  Compare To Zero1 : simulink/Logic and Bit Operations/Compare To Zero  relop=<  OutDataTypeStr=uint8  ZeroCross=off
  Constant : Constant  Value=0
  Constant1 : Constant  Value=UpperLimit
  Constant3 : Constant  Value=LowerLimit
  Discrete-Time Integrator : DiscreteIntegrator  IntegratorMethod=Integration: Trapezoidal  InitialCondition=Init  SampleTime=Ts  LimitOutput=on  UpperSaturationLimit=UpperLimit  LowerSaturationLimit=LowerLimit  ShowStatePort=on  ICPrevOutput=DiscIntNeverNeededParam  ICPrevScaledInput=DiscIntNeverNeededParam
  Kp4 : Gain  Gain=Kp  SaturateOnIntegerOverflow=on  SampleTime=Ts  OutDataTypeStr=Inherit: Same as input  ParamDataTypeStr=Inherit: Same as input
  Kp5 : Gain  Gain=Ki  SaturateOnIntegerOverflow=on  SampleTime=Ts  OutDataTypeStr=Inherit: Same as input  ParamDataTypeStr=Inherit: Same as input
  Logical Operator : Logic  AllPortsSameDT=off  OutDataTypeStr=boolean
  Logical Operator1 : Logic  AllPortsSameDT=off  OutDataTypeStr=boolean
  Logical Operator2 : Logic  Operator=OR  AllPortsSameDT=off  OutDataTypeStr=boolean
  Relational Operator : RelationalOperator  OutDataTypeStr=boolean  InputSameDT=off
  Relational Operator1 : RelationalOperator  Operator=<=  OutDataTypeStr=boolean  InputSameDT=off
  Saturation2 : Saturate  UpperLimit=UpperLimit  LowerLimit=LowerLimit  SampleTime=Ts
  Sum1 : Sum  InputSameDT=on  SaturateOnIntegerOverflow=on  SampleTime=Ts  OutDataTypeStr=Inherit: Same as first input
  Sum6 : Sum  InputSameDT=on  SaturateOnIntegerOverflow=on  SampleTime=Ts  OutDataTypeStr=Inherit: Same as first input
  Switch : Switch  Criteria=u2 > Threshold  SaturateOnIntegerOverflow=off  InputSameDT=off
  Zero-Order Hold : ZeroOrderHold  SampleTime=Ts
  Out : Outport  SampleTime=Ts  InitialOutput=0
  wires:
  Constant/1 -> Switch/1
  Zero-Order Hold/1 -> Sum1/2, Sum6/1
  Discrete-Time Integrator/State -> Sum1/1
  Sum1/1 -> Relational Operator1/1, Relational Operator/1
  Logical Operator2/1 -> Switch/2
  Relational Operator/1 -> Logical Operator/1  "UpperLimit_is_Reached"
  Relational Operator1/1 -> Logical Operator1/1  "LowerLimit_Is_Reached"
  Constant1/1 -> Relational Operator/2
  Constant3/1 -> Relational Operator1/2
  Compare To Zero/1 -> Logical Operator/2  "Error_is_positive"
  Logical Operator/1 -> Logical Operator2/1
  Logical Operator1/1 -> Logical Operator2/2
  Compare To Zero1/1 -> Logical Operator1/2  "Error_is_negative"
  Error/1 -> Compare To Zero1/1, Compare To Zero/1, Kp4/1, Kp5/1
  Sum6/1 -> Saturation2/1
  Kp4/1 -> Zero-Order Hold/1
  Discrete-Time Integrator/1 -> Sum6/2
  Saturation2/1 -> Out/1
  Switch/1 -> Discrete-Time Integrator/1
  Kp5/1 -> Switch/3

== system GridFormingConverter/Grid-Forming Converter/Controllers/PLL, Measurements and Transformation/PLL (3ph) ==
  abc : Inport  PortDimensions=3  SampleTime=Ts
  U_meas : Inport  Port=2  PortDimensions=1
  Model : Subsystem  AncestorBlock=spsPLL3phModel/Discrete  DialogController=POWERSYS.PowerSysDialog
  Freq : Outport  SampleTime=Ts  VectorParamsAs1DForOutWhenUnconnected=off
  wt : Outport  Port=2  SampleTime=Ts  VectorParamsAs1DForOutWhenUnconnected=off
  wires:
  abc/1 -> Model/1(Vabc)
  Model/1(Freq) -> Freq/1
  Model/2(wt) -> wt/1
  U_meas/1 -> Model/2(U_meas)

== system GridFormingConverter/Grid-Forming Converter/Controllers/PWM Generators & Calculation of number of inserted modules (Nin) and number of blocked module (Nbl)/PWM Gen1 ==
  Uref : Inport
  Add6 : Sum
  Clock1 : DigitalClock  SampleTime=ConvCtrl.Ts
  Data Type Conversion : DataTypeConversion  OutDataTypeStr=double  SaturateOnIntegerOverflow=off  RndMeth=Floor
  Fc1 : Constant  Value=Tc
  Fc2 : Constant  Value=Fc
  Logical Operator2 : Logic  Operator=NOT  AllPortsSameDT=off  OutDataTypeStr=boolean
  Lookup Table1 : Lookup  InputValues=[0 .5 1]  Table=[-1 1 -1]  LookUpMeth=Interpolation-Use End Values  SaturateOnIntegerOverflow=off
  Math Function1 : Math  Operator=rem  SignedPower=on
  Mux6 : Mux  Inputs=2
  Phase_rad1 : Constant  Value=Offset_Cr
  Product2 : Product  RndMeth=Zero
  Relational Operator1 : RelationalOperator  OutDataTypeStr=boolean
  SelectPulses : Selector  InputPortWidth=2*n  IndexOptions=Index vector (dialog)  Indices=SelectPulsesPS  OutputSizes=1
  P : Outport
  Cr : Outport  Port=2
  wires:
  Math Function1/1 -> Product2/1
  Relational Operator1/1 -> Mux6/1, Logical Operator2/1
  Product2/1 -> Lookup Table1/1
  Add6/1 -> Math Function1/1
  Clock1/1 -> Add6/1
  Fc1/1 -> Math Function1/2
  Mux6/1 -> SelectPulses/1
  Logical Operator2/1 -> Mux6/2
  Fc2/1 -> Product2/2
  Phase_rad1/1 -> Add6/2
  Lookup Table1/1 -> Cr/1, Relational Operator1/2
  Uref/1 -> Relational Operator1/1
  SelectPulses/1 -> Data Type Conversion/1
  Data Type Conversion/1 -> P/1

== system GridFormingConverter/Grid-Forming Converter/Controllers/PWM Generators & Calculation of number of inserted modules (Nin) and number of blocked module (Nbl)/PWM Gen2 ==
  Uref : Inport
  Add6 : Sum
  Clock1 : DigitalClock  SampleTime=ConvCtrl.Ts
  Data Type Conversion : DataTypeConversion  OutDataTypeStr=double  SaturateOnIntegerOverflow=off  RndMeth=Floor
  Fc1 : Constant  Value=Tc
  Fc2 : Constant  Value=Fc
  Logical Operator2 : Logic  Operator=NOT  AllPortsSameDT=off  OutDataTypeStr=boolean
  Lookup Table1 : Lookup  InputValues=[0 .5 1]  Table=[-1 1 -1]  LookUpMeth=Interpolation-Use End Values  SaturateOnIntegerOverflow=off
  Math Function1 : Math  Operator=rem  SignedPower=on
  Mux6 : Mux  Inputs=2
  Phase_rad1 : Constant  Value=Offset_Cr
  Product2 : Product  RndMeth=Zero
  Relational Operator1 : RelationalOperator  OutDataTypeStr=boolean
  SelectPulses : Selector  InputPortWidth=2*n  IndexOptions=Index vector (dialog)  Indices=SelectPulsesPS  OutputSizes=1
  P : Outport
  Cr : Outport  Port=2
  wires:
  Data Type Conversion/1 -> P/1
  SelectPulses/1 -> Data Type Conversion/1
  Uref/1 -> Relational Operator1/1
  Lookup Table1/1 -> Relational Operator1/2, Cr/1
  Phase_rad1/1 -> Add6/2
  Fc2/1 -> Product2/2
  Logical Operator2/1 -> Mux6/2
  Mux6/1 -> SelectPulses/1
  Fc1/1 -> Math Function1/2
  Clock1/1 -> Add6/1
  Add6/1 -> Math Function1/1
  Product2/1 -> Lookup Table1/1
  Relational Operator1/1 -> Logical Operator2/1, Mux6/1
  Math Function1/1 -> Product2/1

== system GridFormingConverter/Grid-Forming Converter/Controllers/PWM Generators & Calculation of number of inserted modules (Nin) and number of blocked module (Nbl)/PWM Gen3 ==
  Uref : Inport
  Add6 : Sum
  Clock1 : DigitalClock  SampleTime=ConvCtrl.Ts
  Data Type Conversion : DataTypeConversion  OutDataTypeStr=double  SaturateOnIntegerOverflow=off  RndMeth=Floor
  Fc1 : Constant  Value=Tc
  Fc2 : Constant  Value=Fc
  Logical Operator2 : Logic  Operator=NOT  AllPortsSameDT=off  OutDataTypeStr=boolean
  Lookup Table1 : Lookup  InputValues=[0 .5 1]  Table=[-1 1 -1]  LookUpMeth=Interpolation-Use End Values  SaturateOnIntegerOverflow=off
  Math Function1 : Math  Operator=rem  SignedPower=on
  Mux6 : Mux  Inputs=2
  Phase_rad1 : Constant  Value=Offset_Cr
  Product2 : Product  RndMeth=Zero
  Relational Operator1 : RelationalOperator  OutDataTypeStr=boolean
  SelectPulses : Selector  InputPortWidth=2*n  IndexOptions=Index vector (dialog)  Indices=SelectPulsesPS  OutputSizes=1
  P : Outport
  Cr : Outport  Port=2
  wires:
  Math Function1/1 -> Product2/1
  Relational Operator1/1 -> Mux6/1, Logical Operator2/1
  Product2/1 -> Lookup Table1/1
  Add6/1 -> Math Function1/1
  Clock1/1 -> Add6/1
  Fc1/1 -> Math Function1/2
  Mux6/1 -> SelectPulses/1
  Logical Operator2/1 -> Mux6/2
  Fc2/1 -> Product2/2
  Phase_rad1/1 -> Add6/2
  Lookup Table1/1 -> Cr/1, Relational Operator1/2
  Uref/1 -> Relational Operator1/1
  SelectPulses/1 -> Data Type Conversion/1
  Data Type Conversion/1 -> P/1

== system GridFormingConverter/Grid-Forming Converter/Controllers/PWM Generators & Calculation of number of inserted modules (Nin) and number of blocked module (Nbl)/PWM Gen4 ==
  Uref : Inport
  Add6 : Sum
  Clock1 : DigitalClock  SampleTime=ConvCtrl.Ts
  Data Type Conversion : DataTypeConversion  OutDataTypeStr=double  SaturateOnIntegerOverflow=off  RndMeth=Floor
  Fc1 : Constant  Value=Tc
  Fc2 : Constant  Value=Fc
  Logical Operator2 : Logic  Operator=NOT  AllPortsSameDT=off  OutDataTypeStr=boolean
  Lookup Table1 : Lookup  InputValues=[0 .5 1]  Table=[-1 1 -1]  LookUpMeth=Interpolation-Use End Values  SaturateOnIntegerOverflow=off
  Math Function1 : Math  Operator=rem  SignedPower=on
  Mux6 : Mux  Inputs=2
  Phase_rad1 : Constant  Value=Offset_Cr
  Product2 : Product  RndMeth=Zero
  Relational Operator1 : RelationalOperator  OutDataTypeStr=boolean
  SelectPulses : Selector  InputPortWidth=2*n  IndexOptions=Index vector (dialog)  Indices=SelectPulsesPS  OutputSizes=1
  P : Outport
  Cr : Outport  Port=2
  wires:
  Data Type Conversion/1 -> P/1
  SelectPulses/1 -> Data Type Conversion/1
  Uref/1 -> Relational Operator1/1
  Lookup Table1/1 -> Relational Operator1/2, Cr/1
  Phase_rad1/1 -> Add6/2
  Fc2/1 -> Product2/2
  Logical Operator2/1 -> Mux6/2
  Mux6/1 -> SelectPulses/1
  Fc1/1 -> Math Function1/2
  Clock1/1 -> Add6/1
  Add6/1 -> Math Function1/1
  Product2/1 -> Lookup Table1/1
  Relational Operator1/1 -> Logical Operator2/1, Mux6/1
  Math Function1/1 -> Product2/1

== system GridFormingConverter/Grid-Forming Converter/Controllers/PWM Generators & Calculation of number of inserted modules (Nin) and number of blocked module (Nbl)/PWM Gen5 ==
  Uref : Inport
  Add6 : Sum
  Clock1 : DigitalClock  SampleTime=ConvCtrl.Ts
  Data Type Conversion : DataTypeConversion  OutDataTypeStr=double  SaturateOnIntegerOverflow=off  RndMeth=Floor
  Fc1 : Constant  Value=Tc
  Fc2 : Constant  Value=Fc
  Logical Operator2 : Logic  Operator=NOT  AllPortsSameDT=off  OutDataTypeStr=boolean
  Lookup Table1 : Lookup  InputValues=[0 .5 1]  Table=[-1 1 -1]  LookUpMeth=Interpolation-Use End Values  SaturateOnIntegerOverflow=off
  Math Function1 : Math  Operator=rem  SignedPower=on
  Mux6 : Mux  Inputs=2
  Phase_rad1 : Constant  Value=Offset_Cr
  Product2 : Product  RndMeth=Zero
  Relational Operator1 : RelationalOperator  OutDataTypeStr=boolean
  SelectPulses : Selector  InputPortWidth=2*n  IndexOptions=Index vector (dialog)  Indices=SelectPulsesPS  OutputSizes=1
  P : Outport
  Cr : Outport  Port=2
  wires:
  Math Function1/1 -> Product2/1
  Relational Operator1/1 -> Mux6/1, Logical Operator2/1
  Product2/1 -> Lookup Table1/1
  Add6/1 -> Math Function1/1
  Clock1/1 -> Add6/1
  Fc1/1 -> Math Function1/2
  Mux6/1 -> SelectPulses/1
  Logical Operator2/1 -> Mux6/2
  Fc2/1 -> Product2/2
  Phase_rad1/1 -> Add6/2
  Lookup Table1/1 -> Cr/1, Relational Operator1/2
  Uref/1 -> Relational Operator1/1
  SelectPulses/1 -> Data Type Conversion/1
  Data Type Conversion/1 -> P/1

== system GridFormingConverter/Grid-Forming Converter/Controllers/PWM Generators & Calculation of number of inserted modules (Nin) and number of blocked module (Nbl)/PWM Gen6 ==
  Uref : Inport
  Add6 : Sum
  Clock1 : DigitalClock  SampleTime=Ts
  Data Type Conversion : DataTypeConversion  OutDataTypeStr=double  SaturateOnIntegerOverflow=off  RndMeth=Floor
  Fc1 : Constant  Value=Tc
  Fc2 : Constant  Value=Fc
  Logical Operator2 : Logic  Operator=NOT  AllPortsSameDT=off  OutDataTypeStr=boolean
  Lookup Table1 : Lookup  InputValues=[0 .5 1]  Table=[-1 1 -1]  LookUpMeth=Interpolation-Use End Values  SaturateOnIntegerOverflow=off
  Math Function1 : Math  Operator=rem  SignedPower=on
  Mux6 : Mux  Inputs=2
  Phase_rad1 : Constant  Value=Offset_Cr
  Product2 : Product  RndMeth=Zero
  Relational Operator1 : RelationalOperator  OutDataTypeStr=boolean
  SelectPulses : Selector  InputPortWidth=2*n  IndexOptions=Index vector (dialog)  Indices=SelectPulsesPS  OutputSizes=1
  P : Outport
  Cr : Outport  Port=2
  wires:
  Data Type Conversion/1 -> P/1
  SelectPulses/1 -> Data Type Conversion/1
  Uref/1 -> Relational Operator1/1
  Lookup Table1/1 -> Relational Operator1/2, Cr/1
  Phase_rad1/1 -> Add6/2
  Fc2/1 -> Product2/2
  Logical Operator2/1 -> Mux6/2
  Mux6/1 -> SelectPulses/1
  Fc1/1 -> Math Function1/2
  Clock1/1 -> Add6/1
  Add6/1 -> Math Function1/1
  Product2/1 -> Lookup Table1/1
  Relational Operator1/1 -> Logical Operator2/1, Mux6/1
  Math Function1/1 -> Product2/1
